simulink model "robot_controller_m_func"  (R2014a)
settings: Solver=ode45  StartTime=0.0  StopTime=t_final  RelTol=1e-3
values from neighbouring files (symbols this model uses):
  psi0 = 0    [CT_setup.m]    (also in plot_two_kanayama.m)
  vx_disturb = 0    [CT_setup.m]    (also in plot_two_kanayama.m)
  vy_disturb = 0    [CT_setup.m]    (also in plot_two_kanayama.m)
  w_max = 0.25    [CT_setup.m]    (also in plot_two_kanayama.m)
  w_min = -w_max    (= -0.25)    [CT_setup.m]    (also in plot_two_kanayama.m)
  x0 = 0    [CT_setup.m]    (also in plot_two_kanayama.m)
  y0 = 0    [CT_setup.m]    (also in plot_two_kanayama.m)
undefined symbols (not defined in the file or in its folder): UAV_Dynamics, UAV_with_lowlevelcontrol
libraries: simulink x1
settings Model: Creator=user  LastModifiedBy=ysKang
settings DataIOCC: SignalLoggingSaveFormat=ModelDataLogs
settings OptimizationCC: ExpressionDepthLimit=2147483647  InitFltsAndDblsToZero=on
settings DebuggingCC: UnderspecifiedInitializationDetection=Classic  FcnCallInpInsideContextMsg=UseLocalSettings  StateNameClashWarn=warning
settings GRTTargetCC: CombineOutputUpdateFcns=off  GRTInterface=on

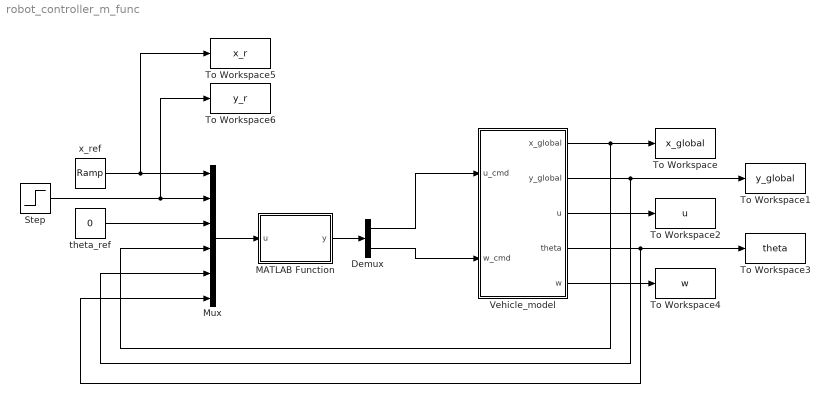
== system robot_controller_m_func ==
  Demux : Demux  Outputs=2
  MATLAB Function : MATLAB Function  TreatAsAtomicUnit=on
  Mux : Mux  Inputs=6
  Step : Step  Time=5  SampleTime=0
  To Workspace : ToWorkspace  VariableName=x_global  SampleTime=-1
  To Workspace1 : ToWorkspace  VariableName=y_global  SampleTime=-1
  To Workspace2 : ToWorkspace  VariableName=u  SampleTime=-1
  To Workspace3 : ToWorkspace  VariableName=theta  SampleTime=-1
  To Workspace4 : ToWorkspace  VariableName=w  SampleTime=-1
  To Workspace5 : ToWorkspace  VariableName=x_r  SampleTime=-1
  To Workspace6 : ToWorkspace  VariableName=y_r  SampleTime=-1
  Vehicle_model : Subsystem  AncestorBlock=UAV_Dynamics/UAV_with_lowlevelcontrol
  theta_ref : Constant  Value=0
  x_ref : simulink/Sources/Ramp  slope=1  start=0  X0=0
  wires:
  Vehicle_model/1(x_global) -> To Workspace/1, Mux/4
  Vehicle_model/2(y_global) -> To Workspace1/1, Mux/5
  Vehicle_model/3(u) -> To Workspace2/1
  Vehicle_model/4(theta) -> To Workspace3/1, Mux/6
  Vehicle_model/5(w) -> To Workspace4/1
  x_ref/1 -> Mux/1, To Workspace5/1
  Step/1 -> Mux/2, To Workspace6/1
  theta_ref/1 -> Mux/3
  Mux/1 -> MATLAB Function/1(u)
  MATLAB Function/1(y) -> Demux/1
  Demux/1 -> Vehicle_model/1(u_cmd)
  Demux/2 -> Vehicle_model/2(w_cmd)

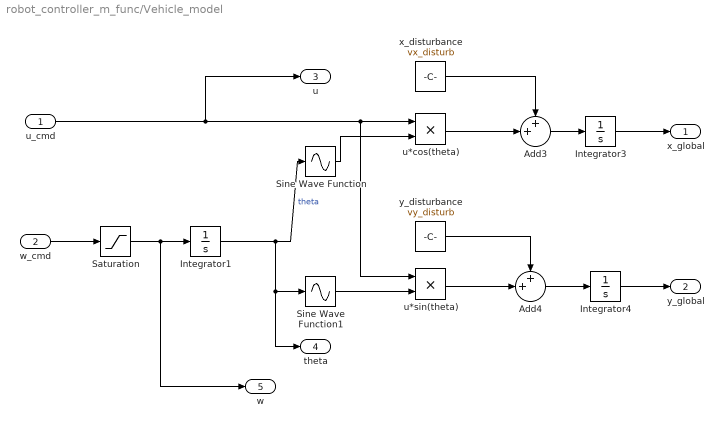
== system robot_controller_m_func/Vehicle_model ==
  u_cmd : Inport
  w_cmd : Inport  Port=2
  Add3 : Sum  Inputs=++|
  Add4 : Sum  Inputs=++|
  Integrator1 : Integrator  InitialCondition=psi0
  Integrator3 : Integrator  InitialCondition=x0
  Integrator4 : Integrator  InitialCondition=y0
  Saturation : Saturate  UpperLimit=w_max  LowerLimit=w_min
  Sine Wave Function : Sin  TimeSource=Use external signal  Phase=pi/2  SampleTime=0
  Sine Wave Function1 : Sin  TimeSource=Use external signal  SampleTime=0
  u*cos(theta) : Product  RndMeth=Zero
  u*sin(theta) : Product  RndMeth=Zero
  x_disturbance : Constant  Value=vx_disturb
  y_disturbance : Constant  Value=vy_disturb
  x_global : Outport
  y_global : Outport  Port=2
  u : Outport  Port=3
  theta : Outport  Port=4
  w : Outport  Port=5
  wires:
  Add4/1 -> Integrator4/1
  u*sin(theta)/1 -> Add4/2
  y_disturbance/1 -> Add4/1
  Add3/1 -> Integrator3/1
  u*cos(theta)/1 -> Add3/2
  x_disturbance/1 -> Add3/1
  Integrator4/1 -> y_global/1
  Integrator3/1 -> x_global/1
  Saturation/1 -> w/1, Integrator1/1
  Integrator1/1 -> Sine Wave Function/1, Sine Wave Function1/1, theta/1  "theta"
  Sine Wave Function/1 -> u*cos(theta)/2
  Sine Wave Function1/1 -> u*sin(theta)/2
  u_cmd/1 -> u*cos(theta)/1, u*sin(theta)/1, u/1
  w_cmd/1 -> Saturation/1

== matlab function robot_controller_m_func/MATLAB Function ==
  data: u input size=6; y output size=2
function y = fcn(u)
%#codegen

Kx = 1;
Ky = 1;
Ktheta = 1;

% Input values
x_r = u(1);
y_r = u(2);
theta_r = u(3);

p_r = [x_r; y_r; theta_r];

x_c = u(4);
y_c = u(5);
theta_c = u(6);

p_c = [x_c; y_c; theta_c];

% Te computation
T_e = [cos(theta_c), sin(theta_c), 0;
    -sin(theta_c), cos(theta_c), 0;
    0, 0, 1];

p_e = T_e*(p_r - p_c);

x_e = p_e(1);
y_e = p_e(2);
theta_e = p_e(3);

% Control Input Computation
v_c = Kx*x_e;
w_c = Ky*y_e + Ktheta*sin(theta_e);

% output values
y = [v_c; w_c];
